simulink model "testing_product_vectors"  (Simulink 7.5)
settings: Solver=ode45  StartTime=0.0  StopTime=10.0  RelTol=1e-3
settings Model: Creator=konstantinos  LastModifiedBy=konstantinos

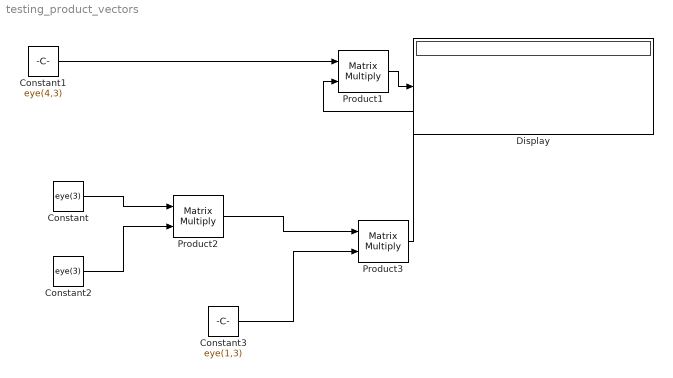
== system testing_product_vectors ==
  Constant : Constant  Value=eye(3)  OutDataType=fixdt(1, 16)  OutScaling=2^0
  Constant1 : Constant  Value=eye(4,3)  OutDataType=fixdt(1, 16)  OutScaling=2^0
  Constant2 : Constant  Value=eye(3)  OutDataType=fixdt(1, 16)  OutScaling=2^0
  Constant3 : Constant  Value=eye(1,3)  OutDataType=fixdt(1, 16)  OutScaling=2^0
  Display : Display
  Product1 : Product  Multiplication=Matrix(*)  OutDataType=fixdt(1, 16)  OutScaling=2^0  RndMeth=Zero
  Product2 : Product  Multiplication=Matrix(*)  OutDataType=fixdt(1, 16)  OutScaling=2^0  RndMeth=Zero
  Product3 : Product  Multiplication=Matrix(*)  OutDataType=fixdt(1, 16)  OutScaling=2^0  RndMeth=Zero
  wires:
  Constant1/1 -> Product1/1
  Product1/1 -> Display/1
  Constant/1 -> Product2/1
  Constant2/1 -> Product2/2
  Product2/1 -> Product3/1
  Product3/1 -> Product1/2
  Constant3/1 -> Product3/2
